simulink model "apcex3"  (Simulink 3.00)
settings: Solver=ode45  SolverMode=SingleTasking  StartTime=0.0  StopTime=10  RelTol=1e-3  AbsTol=1e-6
settings Model: OptimizeBlockIOStorage=off

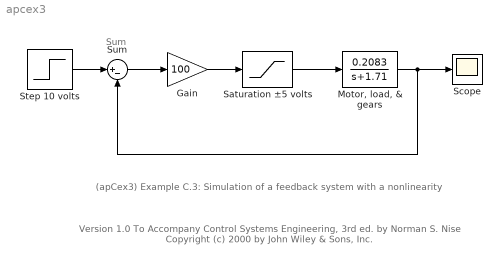
== system apcex3 ==
  note: Sum
  note: (apCex3) Example C.3: Simulation of a feedback system with a nonlinearity
  note: Version 1.0
      | To Accompany Control Systems Engineering, 3rd ed. by Norman S. Nise
      | Copyright (c) 2000 by John Wiley & Sons, Inc.
  Gain : Gain  Gain=100  SaturateOnIntegerOverflow=on
  "Motor, load, & gears" : TransferFcn  Numerator=0.2083  Denominator=[1 1.71]
  "Saturation ±5 volts " : Saturate  UpperLimit=5  LowerLimit=-5
  Scope : Scope
      settings: TickLabels=on  TimeRange=auto  YMin=0  YMax=1.5  SaveToWorkspace=off  SaveName=ScopeData  DataFormat=Matrix
  Step 10 volts : Step  Time=0  Before=0  After=10  SampleTime=-1
  Sum : Sum  Inputs=|+-  SaturateOnIntegerOverflow=on
  wires:
  "Saturation ±5 volts "/1 -> "Motor, load, & gears"/1
  Step 10 volts/1 -> Sum/1
  Sum/1 -> Gain/1
  Gain/1 -> "Saturation ±5 volts "/1
  "Motor, load, & gears"/1 -> Scope/1, Sum/2
